simulink model "sampleModel7293_pp_1_1"  (R2018a)
settings: Solver=VariableStepAuto  StartTime=0.0  StopTime=10.0  RelTol=1e-3
undefined symbols (not defined in the file): DiscIntNeverNeededParam
libraries: simulink x367
(part 4 of 9)

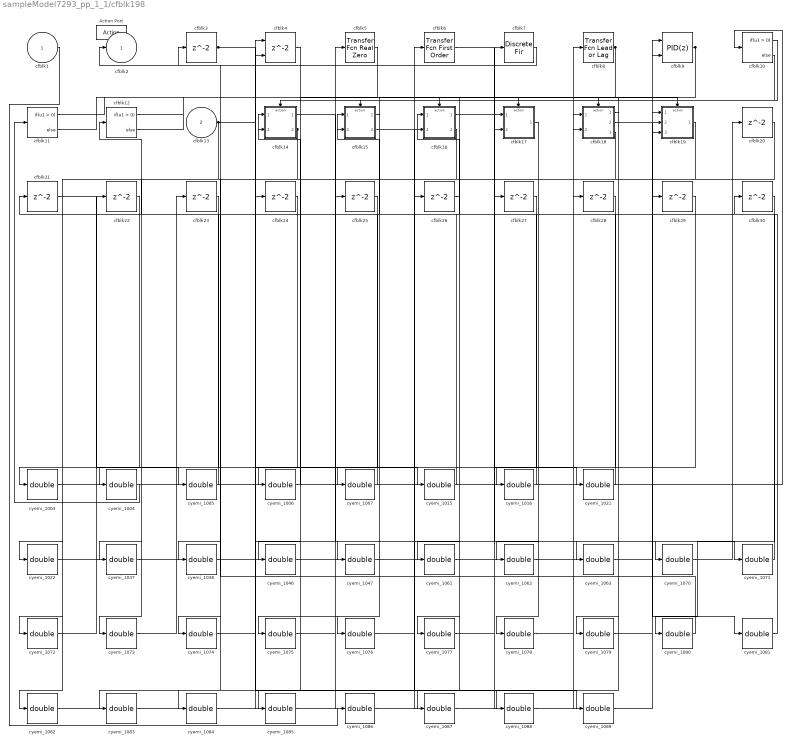
== system sampleModel7293_pp_1_1/cfblk198 ==
  cfblk1 : Inport
  cfblk13 : Inport  Port=2
  Action Port : ActionPort  ActionType=then
  cfblk10 : If  SampleTime=1
  cfblk11 : If  SampleTime=1
  cfblk12 : If  SampleTime=1
  cfblk14 : Subsystem  TreatAsAtomicUnit=on
  cfblk15 : Subsystem  TreatAsAtomicUnit=on
  cfblk16 : Subsystem  TreatAsAtomicUnit=on
  cfblk17 : Subsystem  TreatAsAtomicUnit=on
  cfblk18 : Subsystem  TreatAsAtomicUnit=on
  cfblk19 : Subsystem  TreatAsAtomicUnit=on
  cfblk{3,20..30} (12 alike) : Delay
  cfblk4 : Delay  ShowEnablePort=on
      settings: InputPortMap=u0,e6
  cfblk5 : simulink/Discrete/Transfer Fcn Real Zero  ZeroZ=0.75  ICPrevInput=0.0  DoSatur=off
      settings: SourceProductName=Simulink  SourceProductBaseCode=SL
  cfblk6 : simulink/Discrete/Transfer Fcn First Order  PoleZ=0.95  ICPrevOutput=0.0  DoSatur=off
      settings: SourceProductName=Simulink
  cfblk7 : DiscreteFir
  cfblk8 : simulink/Discrete/Transfer Fcn Lead or Lag  PoleZ=0.95  ZeroZ=0.75  ICPrevOutput=0.0  ICPrevInput=0.0  DoSatur=off
      settings: SourceProductName=Simulink  SourceProductBaseCode=SL
  cfblk9 : simulink/Continuous/PID Controller (2DOF)  Controller=PID  TimeDomain=Discrete-time  SampleTime=-1  IntegratorMethod=Forward Euler  FilterMethod=Forward Euler  Form=Parallel  UseFilter=on  ControllerParametersSource=internal  P=1  I=1  D=0  N=100  b=1  c=1  InitialConditionSource=internal  InitialConditionForIntegrator=0  InitialConditionForFilter=0  ExternalReset=none  LimitOutput=off  UpperSaturationLimit=inf  LowerSaturationLimit=-inf  LinearizeAsGain=off  AntiWindupMode=none  Kb=1  TrackingMode=off  Kt=1  PParamMin=[]  PParamMax=[]  IParamMin=[]  IParamMax=[]  DParamMin=[]  DParamMax=[]  NParamMin=[]  NParamMax=[]  bParamMin=[]  bParamMax=[]  cParamMin=[]  cParamMax=[]  KbParamMin=[]  KbParamMax=[]  KtParamMin=[]  KtParamMax=[]  POutMin=[]  POutMax=[]  IOutMin=[]  IOutMax=[]  DOutMin=[]  DOutMax=[]  NOutMin=[]  NOutMax=[]  bOutMin=[]  bOutMax=[]  cOutMin=[]  cOutMax=[]  KbOutMin=[]  KbOutMax=[]  KtOutMin=[]  KtOutMax=[]  IntegratorOutMin=[]  IntegratorOutMax=[]  FilterOutMin=[]  FilterOutMax=[]  SumOutMin=[]  SumOutMax=[]  Sum1OutMin=[]  Sum1OutMax=[]  Sum2OutMin=[]  Sum2OutMax=[]  Sum3OutMin=[]  Sum3OutMax=[]  SumI1OutMin=[]  SumI1OutMax=[]  SumI2OutMin=[]  SumI2OutMax=[]  SumI3OutMin=[]  SumI3OutMax=[]  SumDOutMin=[]  SumDOutMax=[]  SaturationOutMin=[]  SaturationOutMax=[]  IntegratorContinuousStateAttributes=''  IntegratorStateMustResolveToSignalObject=off  IntegratorRTWStateStorageClass=Auto  FilterContinuousStateAttributes=''  FilterStateMustResolveToSignalObject=off  FilterRTWStateStorageClass=Auto  DifferentiatorICPrevScaledInput=0  DifferentiatorOutMin=[]  DifferentiatorOutMax=[]  FilterDiffOutCoefMin=[]  FilterDiffOutCoefMax=[]  SumDenOutMin=[]  SumDenOutMax=[]  SumNumOutMin=[]  SumNumOutMax=[]  ReciprocalOutMin=[]  ReciprocalOutMax=[]  DivideOutMin=[]  DivideOutMax=[]  TunerSelectOption=Transfer Function Based (PID Tuner App)
  cyemi_{1003..1007,1015..1016,1021..1022,1037..1038,1046..1047,1061..1063,1070..1089} (36 alike) : DataTypeConversion  OutDataTypeStr=double
  cfblk2 : Outport
  wires:
  cfblk7/1 -> cfblk2/1
  cfblk3/1 -> cyemi_1047/1, cyemi_1063/1
  cfblk9/1 -> cyemi_1079/1, cyemi_1087/1
  cfblk13/1 -> cyemi_1004/1, cyemi_1015/1, cyemi_1089/1
  cfblk8/1 -> cyemi_1076/1, cyemi_1077/1
  cfblk14/2(cfblk11) -> cyemi_1073/1, cyemi_1074/1
  cfblk10/1 -> cfblk14/Action
  cfblk10/2 -> cfblk15/Action
  cfblk11/1 -> cfblk16/Action
  cfblk11/2 -> cfblk17/Action
  cfblk12/1 -> cfblk18/Action
  cfblk12/2 -> cfblk19/Action
  cyemi_1003/1 -> cfblk10/1
  cfblk24/1 -> cyemi_1003/1
  cyemi_1004/1 -> cfblk11/1
  cyemi_1005/1 -> cfblk12/1
  cfblk21/1 -> cyemi_1005/1
  cyemi_1006/1 -> cfblk14/1(cfblk1)
  cfblk5/1 -> cyemi_1006/1
  cyemi_1007/1 -> cfblk14/2(cfblk10)
  cfblk25/1 -> cyemi_1007/1
  cyemi_1015/1 -> cfblk15/1(cfblk1)
  cyemi_1016/1 -> cfblk15/2(cfblk6)
  cfblk29/1 -> cyemi_1016/1
  cyemi_1021/1 -> cfblk16/1(cfblk1)
  cfblk6/1 -> cyemi_1021/1
  cyemi_1022/1 -> cfblk16/2(cfblk14)
  cfblk23/1 -> cyemi_1022/1
  cyemi_1037/1 -> cfblk17/1(cfblk1)
  cfblk18/3(cfblk16) -> cyemi_1037/1
  cyemi_1038/1 -> cfblk17/2(cfblk10)
  cfblk27/1 -> cyemi_1038/1
  cyemi_1046/1 -> cfblk18/1(cfblk1)
  cfblk20/1 -> cyemi_1046/1
  cyemi_1047/1 -> cfblk18/2(cfblk14)
  cyemi_1061/1 -> cfblk19/1(cfblk1)
  cfblk26/1 -> cyemi_1061/1
  cyemi_1062/1 -> cfblk19/2(cfblk9)
  cfblk28/1 -> cyemi_1062/1
  cyemi_1063/1 -> cfblk19/3(cfblk10)
  cyemi_1070/1 -> cfblk20/1
  cfblk16/1(cfblk2) -> cyemi_1070/1
  cyemi_1071/1 -> cfblk21/1
  cfblk14/1(cfblk2) -> cyemi_1071/1
  cyemi_1072/1 -> cfblk22/1
  cfblk19/1(cfblk2) -> cyemi_1072/1
  cyemi_1073/1 -> cfblk23/1
  cyemi_1074/1 -> cfblk24/1
  cyemi_1075/1 -> cfblk25/1
  cfblk15/1(cfblk2) -> cyemi_1075/1
  cyemi_1076/1 -> cfblk26/1
  cyemi_1077/1 -> cfblk27/1
  cyemi_1078/1 -> cfblk28/1
  cfblk17/1(cfblk2) -> cyemi_1078/1
  cyemi_1079/1 -> cfblk29/1
  cyemi_1080/1 -> cfblk3/1
  cfblk30/1 -> cyemi_1080/1
  cyemi_1081/1 -> cfblk30/1
  cfblk18/2(cfblk15) -> cyemi_1081/1
  cyemi_1082/1 -> cfblk4/1
  cfblk22/1 -> cyemi_1082/1
  cyemi_1083/1 -> cfblk4/2
  cfblk18/1(cfblk2) -> cyemi_1083/1
  cyemi_1084/1 -> cfblk5/1
  cfblk16/2(cfblk15) -> cyemi_1084/1
  cyemi_1085/1 -> cfblk6/1
  cfblk4/1 -> cyemi_1085/1
  cyemi_1086/1 -> cfblk7/1
  cfblk1/1 -> cyemi_1086/1
  cyemi_1087/1 -> cfblk8/1
  cyemi_1088/1 -> cfblk9/1
  cfblk15/2(cfblk7) -> cyemi_1088/1
  cyemi_1089/1 -> cfblk9/2

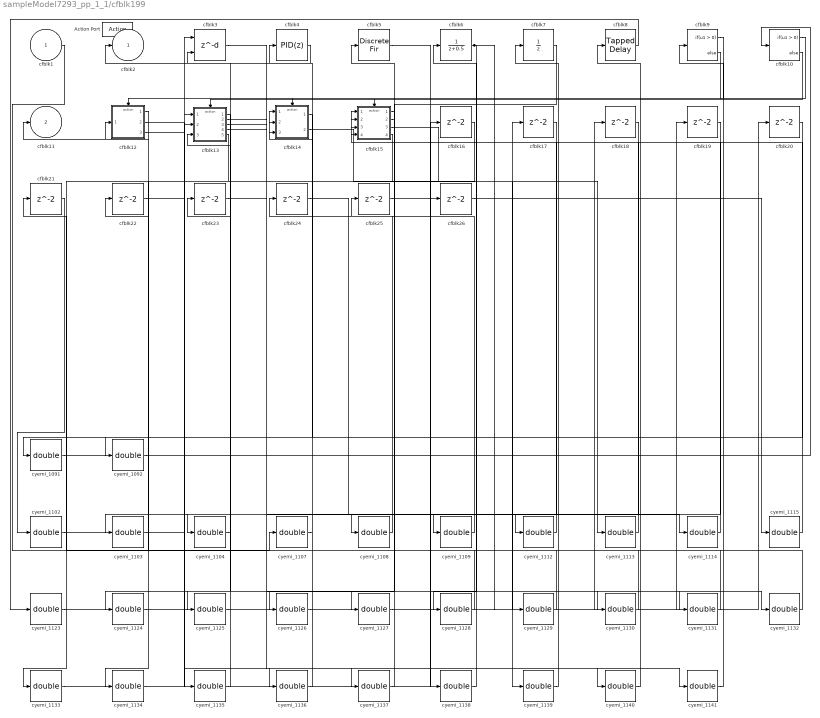
== system sampleModel7293_pp_1_1/cfblk199 ==
  cfblk1 : Inport
  Action Port : ActionPort  ActionType=else
  cfblk10 : If  SampleTime=1
  cfblk12 : Subsystem  TreatAsAtomicUnit=on
  cfblk13 : Subsystem  TreatAsAtomicUnit=on
  cfblk14 : Subsystem  TreatAsAtomicUnit=on
  cfblk15 : Subsystem  TreatAsAtomicUnit=on
  cfblk{16..26} (11 alike) : Delay
  cfblk3 : Delay  DelayLengthSource=Input port
      settings: InputPortMap=u0,p1
  cfblk4 : simulink/Continuous/PID Controller  Controller=PID  TimeDomain=Discrete-time  SampleTime=-1  IntegratorMethod=Forward Euler  FilterMethod=Forward Euler  Form=Parallel  UseFilter=on  ControllerParametersSource=internal  P=1  I=1  D=0  N=100  InitialConditionSource=internal  InitialConditionForIntegrator=0  InitialConditionForFilter=0  ExternalReset=none  LimitOutput=off  UpperSaturationLimit=inf  LowerSaturationLimit=-inf  LinearizeAsGain=off  AntiWindupMode=none  Kb=1  TrackingMode=off  Kt=1  PParamMin=[]  PParamMax=[]  IParamMin=[]  IParamMax=[]  DParamMin=[]  DParamMax=[]  NParamMin=[]  NParamMax=[]  KbParamMin=[]  KbParamMax=[]  KtParamMin=[]  KtParamMax=[]  POutMin=[]  POutMax=[]  IOutMin=[]  IOutMax=[]  DOutMin=[]  DOutMax=[]  NOutMin=[]  NOutMax=[]  KbOutMin=[]  KbOutMax=[]  KtOutMin=[]  KtOutMax=[]  IntegratorOutMin=[]  IntegratorOutMax=[]  FilterOutMin=[]  FilterOutMax=[]  SumOutMin=[]  SumOutMax=[]  SumI1OutMin=[]  SumI1OutMax=[]  SumI2OutMin=[]  SumI2OutMax=[]  SumI3OutMin=[]  SumI3OutMax=[]  SumDOutMin=[]  SumDOutMax=[]  SaturationOutMin=[]  SaturationOutMax=[]  IntegratorContinuousStateAttributes=''  IntegratorStateMustResolveToSignalObject=off  IntegratorRTWStateStorageClass=Auto  FilterContinuousStateAttributes=''  FilterStateMustResolveToSignalObject=off  FilterRTWStateStorageClass=Auto  DifferentiatorICPrevScaledInput=0  DifferentiatorOutMin=[]  DifferentiatorOutMax=[]  FilterDiffOutCoefMin=[]  FilterDiffOutCoefMax=[]  SumDenOutMin=[]  SumDenOutMax=[]  SumNumOutMin=[]  SumNumOutMax=[]  ReciprocalOutMin=[]  ReciprocalOutMax=[]  DivideOutMin=[]  DivideOutMax=[]  TunerSelectOption=Transfer Function Based (PID Tuner App)
  cfblk5 : DiscreteFir
  cfblk6 : DiscreteTransferFcn
  cfblk7 : UnitDelay  SampleTime=-1
  cfblk8 : simulink/Discrete/Tapped Delay  vinit=0.0  samptime=-1  NumDelays=1  DelayOrder=Oldest  includeCurrent=off
  cfblk9 : If  SampleTime=1
  cyemi_{1091..1092,1102..1104,1107..1109,1112..1115,1123..1141} (31 alike) : DataTypeConversion  OutDataTypeStr=double
  cfblk2 : Outport
  cfblk11 : Outport  Port=2
  wires:
  cfblk12/1(cfblk2) -> cfblk11/1
  cfblk6/1 -> cyemi_1128/1, cyemi_1129/1
  cfblk4/1 -> cfblk2/1
  cfblk9/1 -> cfblk12/Action
  cfblk9/2 -> cfblk13/Action
  cfblk10/1 -> cfblk14/Action
  cfblk10/2 -> cfblk15/Action
  cyemi_1091/1 -> cfblk10/1
  cfblk20/1 -> cyemi_1091/1
  cyemi_1092/1 -> cfblk12/1(cfblk1)
  cfblk14/1(cfblk2) -> cyemi_1092/1
  cyemi_1102/1 -> cfblk13/1(cfblk1)
  cfblk21/1 -> cyemi_1102/1
  cyemi_1103/1 -> cfblk13/2(cfblk5)
  cfblk18/1 -> cyemi_1103/1
  cyemi_1104/1 -> cfblk13/3(cfblk6)
  cfblk16/1 -> cyemi_1104/1
  cyemi_1107/1 -> cfblk14/1(cfblk1)
  cfblk1/1 -> cyemi_1107/1
  cyemi_1108/1 -> cfblk14/2(cfblk5)
  cfblk23/1 -> cyemi_1108/1
  cyemi_1109/1 -> cfblk14/3(cfblk6)
  cfblk19/1 -> cyemi_1109/1
  cyemi_1112/1 -> cfblk15/1(cfblk1)
  cfblk17/1 -> cyemi_1112/1
  cyemi_1113/1 -> cfblk15/2(cfblk9)
  cfblk14/2(cfblk7) -> cyemi_1113/1
  cyemi_1114/1 -> cfblk15/3(cfblk10)
  cfblk24/1 -> cyemi_1114/1
  cyemi_1115/1 -> cfblk15/4(cfblk11)
  cfblk26/1 -> cyemi_1115/1
  cyemi_1123/1 -> cfblk16/1
  cfblk8/1 -> cyemi_1123/1
  cyemi_1124/1 -> cfblk17/1
  cfblk13/1(cfblk2) -> cyemi_1124/1
  cyemi_1125/1 -> cfblk18/1
  cfblk15/1(cfblk2) -> cyemi_1125/1
  cyemi_1126/1 -> cfblk19/1
  cfblk15/2(cfblk12) -> cyemi_1126/1
  cyemi_1127/1 -> cfblk20/1
  cfblk7/1 -> cyemi_1127/1
  cyemi_1128/1 -> cfblk21/1
  cyemi_1129/1 -> cfblk22/1
  cyemi_1130/1 -> cfblk23/1
  cfblk13/2(cfblk7) -> cyemi_1130/1
  cyemi_1131/1 -> cfblk24/1
  cfblk13/3(cfblk8) -> cyemi_1131/1
  cyemi_1132/1 -> cfblk25/1
  cfblk13/4(cfblk9) -> cyemi_1132/1
  cyemi_1133/1 -> cfblk26/1
  cfblk13/5(cfblk10) -> cyemi_1133/1
  cyemi_1134/1 -> cfblk3/1
  cfblk15/4(cfblk14) -> cyemi_1134/1
  cyemi_1135/1 -> cfblk3/2
  cfblk22/1 -> cyemi_1135/1
  cyemi_1136/1 -> cfblk4/1
  cfblk12/2(cfblk9) -> cyemi_1136/1
  cyemi_1137/1 -> cfblk5/1
  cfblk3/1 -> cyemi_1137/1
  cyemi_1138/1 -> cfblk6/1
  cfblk5/1 -> cyemi_1138/1
  cyemi_1139/1 -> cfblk7/1
  cfblk15/3(cfblk13) -> cyemi_1139/1
  cyemi_1140/1 -> cfblk8/1
  cfblk12/3(cfblk10) -> cyemi_1140/1
  cyemi_1141/1 -> cfblk9/1
  cfblk25/1 -> cyemi_1141/1

== system sampleModel7293_pp_1_1/cfblk200 ==
  cfblk1 : Inport
  Action Port : ActionPort  ActionType=then
  cfblk10 : If  SampleTime=1
  cfblk11 : Subsystem  TreatAsAtomicUnit=on
  cfblk12 : Subsystem  TreatAsAtomicUnit=on
  cfblk13 : Delay
  cfblk14 : Delay
  cfblk3 : simulink/Discrete/Tapped Delay  vinit=0.0  samptime=-1  NumDelays=1  DelayOrder=Oldest  includeCurrent=off
  cfblk4 : simulink/Discrete/Difference  ICPrevInput=0.0  OutMin=[]  OutMax=[]  OutDataTypeStr=double  OutputDataTypeScalingMode=double  OutDataType=fixdt(1, 16)  OutScaling=2^-10  DoSatur=off
  cfblk5 : Delay  DelayLengthSource=Input port
      settings: InputPortMap=u0,p1
  cfblk6 : Delay
  cfblk7 : UnitDelay  SampleTime=-1
  cfblk8 : simulink/Continuous/PID Controller (2DOF)  Controller=PID  TimeDomain=Discrete-time  SampleTime=-1  IntegratorMethod=Forward Euler  FilterMethod=Forward Euler  Form=Parallel  UseFilter=on  ControllerParametersSource=internal  P=1  I=1  D=0  N=100  b=1  c=1  InitialConditionSource=internal  InitialConditionForIntegrator=0  InitialConditionForFilter=0  ExternalReset=none  LimitOutput=off  UpperSaturationLimit=inf  LowerSaturationLimit=-inf  LinearizeAsGain=off  AntiWindupMode=none  Kb=1  TrackingMode=off  Kt=1  PParamMin=[]  PParamMax=[]  IParamMin=[]  IParamMax=[]  DParamMin=[]  DParamMax=[]  NParamMin=[]  NParamMax=[]  bParamMin=[]  bParamMax=[]  cParamMin=[]  cParamMax=[]  KbParamMin=[]  KbParamMax=[]  KtParamMin=[]  KtParamMax=[]  POutMin=[]  POutMax=[]  IOutMin=[]  IOutMax=[]  DOutMin=[]  DOutMax=[]  NOutMin=[]  NOutMax=[]  bOutMin=[]  bOutMax=[]  cOutMin=[]  cOutMax=[]  KbOutMin=[]  KbOutMax=[]  KtOutMin=[]  KtOutMax=[]  IntegratorOutMin=[]  IntegratorOutMax=[]  FilterOutMin=[]  FilterOutMax=[]  SumOutMin=[]  SumOutMax=[]  Sum1OutMin=[]  Sum1OutMax=[]  Sum2OutMin=[]  Sum2OutMax=[]  Sum3OutMin=[]  Sum3OutMax=[]  SumI1OutMin=[]  SumI1OutMax=[]  SumI2OutMin=[]  SumI2OutMax=[]  SumI3OutMin=[]  SumI3OutMax=[]  SumDOutMin=[]  SumDOutMax=[]  SaturationOutMin=[]  SaturationOutMax=[]  IntegratorContinuousStateAttributes=''  IntegratorStateMustResolveToSignalObject=off  IntegratorRTWStateStorageClass=Auto  FilterContinuousStateAttributes=''  FilterStateMustResolveToSignalObject=off  FilterRTWStateStorageClass=Auto  DifferentiatorICPrevScaledInput=0  DifferentiatorOutMin=[]  DifferentiatorOutMax=[]  FilterDiffOutCoefMin=[]  FilterDiffOutCoefMax=[]  SumDenOutMin=[]  SumDenOutMax=[]  SumNumOutMin=[]  SumNumOutMax=[]  ReciprocalOutMin=[]  ReciprocalOutMax=[]  DivideOutMin=[]  DivideOutMax=[]  TunerSelectOption=Transfer Function Based (PID Tuner App)
  cfblk9 : UnitDelay  SampleTime=-1
  cyemi_{1145..1146,1157..1158,1169..1179} (15 alike) : DataTypeConversion  OutDataTypeStr=double
  cfblk2 : Outport
  wires:
  cfblk3/1 -> cyemi_1145/1, cyemi_1157/1, cyemi_1178/1
  cfblk9/1 -> cfblk2/1
  cfblk5/1 -> cyemi_1158/1, cyemi_1176/1
  cfblk6/1 -> cyemi_1174/1, cyemi_1179/1
  cfblk10/1 -> cfblk11/Action
  cfblk10/2 -> cfblk12/Action
  cyemi_1145/1 -> cfblk10/1
  cyemi_1146/1 -> cfblk11/1(cfblk1)
  cfblk14/1 -> cyemi_1146/1
  cyemi_1157/1 -> cfblk12/1(cfblk1)
  cyemi_1158/1 -> cfblk12/2(cfblk9)
  cyemi_1169/1 -> cfblk13/1
  cfblk8/1 -> cyemi_1169/1
  cyemi_1170/1 -> cfblk14/1
  cfblk4/1 -> cyemi_1170/1
  cyemi_1171/1 -> cfblk3/1
  cfblk7/1 -> cyemi_1171/1
  cyemi_1172/1 -> cfblk4/1
  cfblk11/1(cfblk2) -> cyemi_1172/1
  cyemi_1173/1 -> cfblk5/1
  cfblk13/1 -> cyemi_1173/1
  cyemi_1174/1 -> cfblk5/2
  cyemi_1175/1 -> cfblk6/1
  cfblk1/1 -> cyemi_1175/1
  cyemi_1176/1 -> cfblk7/1
  cyemi_1177/1 -> cfblk8/1
  cfblk12/1(cfblk2) -> cyemi_1177/1
  cyemi_1178/1 -> cfblk8/2
  cyemi_1179/1 -> cfblk9/1

== system sampleModel7293_pp_1_1/cfblk201 ==
  cfblk1 : Inport
  Action Port : ActionPort  ActionType=else
  cfblk10 : simulink/Discrete/Transfer Fcn First Order  PoleZ=0.95  ICPrevOutput=0.0  DoSatur=off
      settings: SourceProductName=Simulink
  cfblk11 : DiscreteIntegrator  SampleTime=-1  OutDataTypeStr=double  ICPrevOutput=DiscIntNeverNeededParam  ICPrevScaledInput=DiscIntNeverNeededParam
  cfblk12 : DiscreteTransferFcn
  cfblk13 : simulink/Discrete/Transfer Fcn Real Zero  ZeroZ=0.75  ICPrevInput=0.0  DoSatur=off
      settings: SourceProductName=Simulink  SourceProductBaseCode=SL
  cfblk14 : DiscreteStateSpace  SampleTime=-1
  cfblk15 : Delay
  cfblk3 : UnitDelay  SampleTime=-1
  cfblk4 : Delay  DelayLengthSource=Input port
      settings: InputPortMap=u0,p1
  cfblk5 : DiscreteFir
  cfblk6 : DiscreteTransferFcn
  cfblk7 : DiscreteIntegrator  SampleTime=-1  OutDataTypeStr=double  ICPrevOutput=DiscIntNeverNeededParam  ICPrevScaledInput=DiscIntNeverNeededParam
  cfblk8 : DiscreteStateSpace  SampleTime=-1
  cfblk9 : Delay
  cyemi_{1181..1194} (14 alike) : DataTypeConversion  OutDataTypeStr=double
  cfblk2 : Outport
  wires:
  cfblk1/1 -> cyemi_1189/1, cyemi_1190/1
  cfblk13/1 -> cfblk2/1
  cyemi_1181/1 -> cfblk10/1
  cfblk14/1 -> cyemi_1181/1
  cyemi_1182/1 -> cfblk11/1
  cfblk12/1 -> cyemi_1182/1
  cyemi_1183/1 -> cfblk12/1
  cfblk6/1 -> cyemi_1183/1
  cyemi_1184/1 -> cfblk13/1
  cfblk4/1 -> cyemi_1184/1
  cyemi_1185/1 -> cfblk14/1
  cfblk8/1 -> cyemi_1185/1
  cyemi_1186/1 -> cfblk15/1
  cfblk9/1 -> cyemi_1186/1
  cyemi_1187/1 -> cfblk3/1
  cfblk11/1 -> cyemi_1187/1
  cyemi_1188/1 -> cfblk4/1
  cfblk3/1 -> cyemi_1188/1
  cyemi_1189/1 -> cfblk4/2
  cyemi_1190/1 -> cfblk5/1
  cyemi_1191/1 -> cfblk6/1
  cfblk7/1 -> cyemi_1191/1
  cyemi_1192/1 -> cfblk7/1
  cfblk5/1 -> cyemi_1192/1
  cyemi_1193/1 -> cfblk8/1
  cfblk15/1 -> cyemi_1193/1
  cyemi_1194/1 -> cfblk9/1
  cfblk10/1 -> cyemi_1194/1

== system sampleModel7293_pp_1_1/cfblk202 ==
  cfblk1 : Inport
  Action Port : ActionPort  ActionType=then
  cfblk10 : DiscreteStateSpace  SampleTime=-1
  cfblk11 : DiscreteTransferFcn
  cfblk12 : Delay
  cfblk13 : Delay
  cfblk3 : simulink/Discrete/Tapped Delay  vinit=0.0  samptime=-1  NumDelays=1  DelayOrder=Oldest  includeCurrent=off
  cfblk4 : simulink/Discrete/Transfer Fcn Lead or Lag  PoleZ=0.95  ZeroZ=0.75  ICPrevOutput=0.0  ICPrevInput=0.0  DoSatur=off
      settings: SourceProductName=Simulink  SourceProductBaseCode=SL
  cfblk5 : simulink/Continuous/PID Controller (2DOF)  Controller=PID  TimeDomain=Discrete-time  SampleTime=-1  IntegratorMethod=Forward Euler  FilterMethod=Forward Euler  Form=Parallel  UseFilter=on  ControllerParametersSource=internal  P=1  I=1  D=0  N=100  b=1  c=1  InitialConditionSource=internal  InitialConditionForIntegrator=0  InitialConditionForFilter=0  ExternalReset=none  LimitOutput=off  UpperSaturationLimit=inf  LowerSaturationLimit=-inf  LinearizeAsGain=off  AntiWindupMode=none  Kb=1  TrackingMode=off  Kt=1  PParamMin=[]  PParamMax=[]  IParamMin=[]  IParamMax=[]  DParamMin=[]  DParamMax=[]  NParamMin=[]  NParamMax=[]  bParamMin=[]  bParamMax=[]  cParamMin=[]  cParamMax=[]  KbParamMin=[]  KbParamMax=[]  KtParamMin=[]  KtParamMax=[]  POutMin=[]  POutMax=[]  IOutMin=[]  IOutMax=[]  DOutMin=[]  DOutMax=[]  NOutMin=[]  NOutMax=[]  bOutMin=[]  bOutMax=[]  cOutMin=[]  cOutMax=[]  KbOutMin=[]  KbOutMax=[]  KtOutMin=[]  KtOutMax=[]  IntegratorOutMin=[]  IntegratorOutMax=[]  FilterOutMin=[]  FilterOutMax=[]  SumOutMin=[]  SumOutMax=[]  Sum1OutMin=[]  Sum1OutMax=[]  Sum2OutMin=[]  Sum2OutMax=[]  Sum3OutMin=[]  Sum3OutMax=[]  SumI1OutMin=[]  SumI1OutMax=[]  SumI2OutMin=[]  SumI2OutMax=[]  SumI3OutMin=[]  SumI3OutMax=[]  SumDOutMin=[]  SumDOutMax=[]  SaturationOutMin=[]  SaturationOutMax=[]  IntegratorContinuousStateAttributes=''  IntegratorStateMustResolveToSignalObject=off  IntegratorRTWStateStorageClass=Auto  FilterContinuousStateAttributes=''  FilterStateMustResolveToSignalObject=off  FilterRTWStateStorageClass=Auto  DifferentiatorICPrevScaledInput=0  DifferentiatorOutMin=[]  DifferentiatorOutMax=[]  FilterDiffOutCoefMin=[]  FilterDiffOutCoefMax=[]  SumDenOutMin=[]  SumDenOutMax=[]  SumNumOutMin=[]  SumNumOutMax=[]  ReciprocalOutMin=[]  ReciprocalOutMax=[]  DivideOutMin=[]  DivideOutMax=[]  TunerSelectOption=Transfer Function Based (PID Tuner App)
  cfblk6 : UnitDelay  SampleTime=-1
  cfblk7 : DiscreteFir
  cfblk8 : Delay  DelayLengthSource=Input port
      settings: InputPortMap=u0,p1
  cfblk9 : simulink/Continuous/PID Controller (2DOF)  Controller=PID  TimeDomain=Discrete-time  SampleTime=-1  IntegratorMethod=Forward Euler  FilterMethod=Forward Euler  Form=Parallel  UseFilter=on  ControllerParametersSource=internal  P=1  I=1  D=0  N=100  b=1  c=1  InitialConditionSource=internal  InitialConditionForIntegrator=0  InitialConditionForFilter=0  ExternalReset=none  LimitOutput=off  UpperSaturationLimit=inf  LowerSaturationLimit=-inf  LinearizeAsGain=off  AntiWindupMode=none  Kb=1  TrackingMode=off  Kt=1  PParamMin=[]  PParamMax=[]  IParamMin=[]  IParamMax=[]  DParamMin=[]  DParamMax=[]  NParamMin=[]  NParamMax=[]  bParamMin=[]  bParamMax=[]  cParamMin=[]  cParamMax=[]  KbParamMin=[]  KbParamMax=[]  KtParamMin=[]  KtParamMax=[]  POutMin=[]  POutMax=[]  IOutMin=[]  IOutMax=[]  DOutMin=[]  DOutMax=[]  NOutMin=[]  NOutMax=[]  bOutMin=[]  bOutMax=[]  cOutMin=[]  cOutMax=[]  KbOutMin=[]  KbOutMax=[]  KtOutMin=[]  KtOutMax=[]  IntegratorOutMin=[]  IntegratorOutMax=[]  FilterOutMin=[]  FilterOutMax=[]  SumOutMin=[]  SumOutMax=[]  Sum1OutMin=[]  Sum1OutMax=[]  Sum2OutMin=[]  Sum2OutMax=[]  Sum3OutMin=[]  Sum3OutMax=[]  SumI1OutMin=[]  SumI1OutMax=[]  SumI2OutMin=[]  SumI2OutMax=[]  SumI3OutMin=[]  SumI3OutMax=[]  SumDOutMin=[]  SumDOutMax=[]  SaturationOutMin=[]  SaturationOutMax=[]  IntegratorContinuousStateAttributes=''  IntegratorStateMustResolveToSignalObject=off  IntegratorRTWStateStorageClass=Auto  FilterContinuousStateAttributes=''  FilterStateMustResolveToSignalObject=off  FilterRTWStateStorageClass=Auto  DifferentiatorICPrevScaledInput=0  DifferentiatorOutMin=[]  DifferentiatorOutMax=[]  FilterDiffOutCoefMin=[]  FilterDiffOutCoefMax=[]  SumDenOutMin=[]  SumDenOutMax=[]  SumNumOutMin=[]  SumNumOutMax=[]  ReciprocalOutMin=[]  ReciprocalOutMax=[]  DivideOutMin=[]  DivideOutMax=[]  TunerSelectOption=Transfer Function Based (PID Tuner App)
  cyemi_{1196..1209} (14 alike) : DataTypeConversion  OutDataTypeStr=double
  cfblk2 : Outport
  wires:
  cfblk3/1 -> cyemi_1201/1, cyemi_1203/1, cyemi_1209/1
  cfblk9/1 -> cfblk2/1
  cfblk11/1 -> cyemi_1199/1, cyemi_1202/1
  cyemi_1196/1 -> cfblk10/1
  cfblk1/1 -> cyemi_1196/1
  cyemi_1197/1 -> cfblk11/1
  cfblk6/1 -> cyemi_1197/1
  cyemi_1198/1 -> cfblk12/1
  cfblk4/1 -> cyemi_1198/1
  cyemi_1199/1 -> cfblk13/1
  cyemi_1200/1 -> cfblk3/1
  cfblk12/1 -> cyemi_1200/1
  cyemi_1201/1 -> cfblk4/1
  cyemi_1202/1 -> cfblk5/1
  cyemi_1203/1 -> cfblk5/2
  cyemi_1204/1 -> cfblk6/1
  cfblk13/1 -> cyemi_1204/1
  cyemi_1205/1 -> cfblk7/1
  cfblk10/1 -> cyemi_1205/1
  cyemi_1206/1 -> cfblk8/1
  cfblk5/1 -> cyemi_1206/1
  cyemi_1207/1 -> cfblk8/2
  cfblk7/1 -> cyemi_1207/1
  cyemi_1208/1 -> cfblk9/1
  cfblk8/1 -> cyemi_1208/1
  cyemi_1209/1 -> cfblk9/2

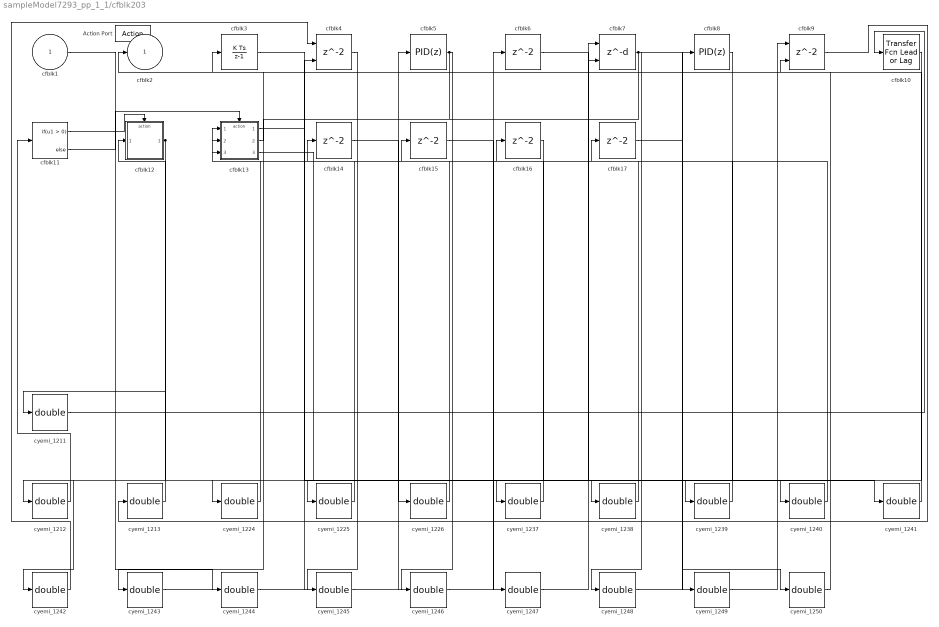
== system sampleModel7293_pp_1_1/cfblk203 ==
  cfblk1 : Inport
  Action Port : ActionPort  ActionType=else
  cfblk10 : simulink/Discrete/Transfer Fcn Lead or Lag  PoleZ=0.95  ZeroZ=0.75  ICPrevOutput=0.0  ICPrevInput=0.0  DoSatur=off
      settings: SourceProductName=Simulink  SourceProductBaseCode=SL
  cfblk11 : If  SampleTime=1
  cfblk12 : Subsystem  TreatAsAtomicUnit=on
  cfblk13 : Subsystem  TreatAsAtomicUnit=on
  cfblk{6,14..17} (5 alike) : Delay
  cfblk3 : DiscreteIntegrator  SampleTime=-1  OutDataTypeStr=double  ICPrevOutput=DiscIntNeverNeededParam  ICPrevScaledInput=DiscIntNeverNeededParam
  cfblk4 : Delay  ShowEnablePort=on
      settings: InputPortMap=u0,e6
  cfblk5 : simulink/Continuous/PID Controller  Controller=PID  TimeDomain=Discrete-time  SampleTime=-1  IntegratorMethod=Forward Euler  FilterMethod=Forward Euler  Form=Parallel  UseFilter=on  ControllerParametersSource=internal  P=1  I=1  D=0  N=100  InitialConditionSource=internal  InitialConditionForIntegrator=0  InitialConditionForFilter=0  ExternalReset=none  LimitOutput=off  UpperSaturationLimit=inf  LowerSaturationLimit=-inf  LinearizeAsGain=off  AntiWindupMode=none  Kb=1  TrackingMode=off  Kt=1  PParamMin=[]  PParamMax=[]  IParamMin=[]  IParamMax=[]  DParamMin=[]  DParamMax=[]  NParamMin=[]  NParamMax=[]  KbParamMin=[]  KbParamMax=[]  KtParamMin=[]  KtParamMax=[]  POutMin=[]  POutMax=[]  IOutMin=[]  IOutMax=[]  DOutMin=[]  DOutMax=[]  NOutMin=[]  NOutMax=[]  KbOutMin=[]  KbOutMax=[]  KtOutMin=[]  KtOutMax=[]  IntegratorOutMin=[]  IntegratorOutMax=[]  FilterOutMin=[]  FilterOutMax=[]  SumOutMin=[]  SumOutMax=[]  SumI1OutMin=[]  SumI1OutMax=[]  SumI2OutMin=[]  SumI2OutMax=[]  SumI3OutMin=[]  SumI3OutMax=[]  SumDOutMin=[]  SumDOutMax=[]  SaturationOutMin=[]  SaturationOutMax=[]  IntegratorContinuousStateAttributes=''  IntegratorStateMustResolveToSignalObject=off  IntegratorRTWStateStorageClass=Auto  FilterContinuousStateAttributes=''  FilterStateMustResolveToSignalObject=off  FilterRTWStateStorageClass=Auto  DifferentiatorICPrevScaledInput=0  DifferentiatorOutMin=[]  DifferentiatorOutMax=[]  FilterDiffOutCoefMin=[]  FilterDiffOutCoefMax=[]  SumDenOutMin=[]  SumDenOutMax=[]  SumNumOutMin=[]  SumNumOutMax=[]  ReciprocalOutMin=[]  ReciprocalOutMax=[]  DivideOutMin=[]  DivideOutMax=[]  TunerSelectOption=Transfer Function Based (PID Tuner App)
  cfblk7 : Delay  DelayLengthSource=Input port
      settings: InputPortMap=u0,p1
  cfblk8 : simulink/Continuous/PID Controller  Controller=PID  TimeDomain=Discrete-time  SampleTime=-1  IntegratorMethod=Forward Euler  FilterMethod=Forward Euler  Form=Parallel  UseFilter=on  ControllerParametersSource=internal  P=1  I=1  D=0  N=100  InitialConditionSource=internal  InitialConditionForIntegrator=0  InitialConditionForFilter=0  ExternalReset=none  LimitOutput=off  UpperSaturationLimit=inf  LowerSaturationLimit=-inf  LinearizeAsGain=off  AntiWindupMode=none  Kb=1  TrackingMode=off  Kt=1  PParamMin=[]  PParamMax=[]  IParamMin=[]  IParamMax=[]  DParamMin=[]  DParamMax=[]  NParamMin=[]  NParamMax=[]  KbParamMin=[]  KbParamMax=[]  KtParamMin=[]  KtParamMax=[]  POutMin=[]  POutMax=[]  IOutMin=[]  IOutMax=[]  DOutMin=[]  DOutMax=[]  NOutMin=[]  NOutMax=[]  KbOutMin=[]  KbOutMax=[]  KtOutMin=[]  KtOutMax=[]  IntegratorOutMin=[]  IntegratorOutMax=[]  FilterOutMin=[]  FilterOutMax=[]  SumOutMin=[]  SumOutMax=[]  SumI1OutMin=[]  SumI1OutMax=[]  SumI2OutMin=[]  SumI2OutMax=[]  SumI3OutMin=[]  SumI3OutMax=[]  SumDOutMin=[]  SumDOutMax=[]  SaturationOutMin=[]  SaturationOutMax=[]  IntegratorContinuousStateAttributes=''  IntegratorStateMustResolveToSignalObject=off  IntegratorRTWStateStorageClass=Auto  FilterContinuousStateAttributes=''  FilterStateMustResolveToSignalObject=off  FilterRTWStateStorageClass=Auto  DifferentiatorICPrevScaledInput=0  DifferentiatorOutMin=[]  DifferentiatorOutMax=[]  FilterDiffOutCoefMin=[]  FilterDiffOutCoefMax=[]  SumDenOutMin=[]  SumDenOutMax=[]  SumNumOutMin=[]  SumNumOutMax=[]  ReciprocalOutMin=[]  ReciprocalOutMax=[]  DivideOutMin=[]  DivideOutMax=[]  TunerSelectOption=Transfer Function Based (PID Tuner App)
  cfblk9 : Delay  ShowEnablePort=on
      settings: InputPortMap=u0,e6
  cyemi_{1211..1213,1224..1226,1237..1250} (20 alike) : DataTypeConversion  OutDataTypeStr=double
  cfblk2 : Outport
  wires:
  cfblk5/1 -> cyemi_1212/1, cyemi_1246/1
  cfblk12/1(cfblk2) -> cyemi_1211/1, cyemi_1242/1
  cfblk7/1 -> cyemi_1243/1, cyemi_1248/1, cyemi_1250/1
  cfblk13/2(cfblk14) -> cfblk2/1
  cfblk11/1 -> cfblk12/Action
  cfblk11/2 -> cfblk13/Action
  cyemi_1211/1 -> cfblk10/1
  cyemi_1212/1 -> cfblk11/1
  cyemi_1213/1 -> cfblk12/1(cfblk1)
  cfblk9/1 -> cyemi_1213/1
  cyemi_1224/1 -> cfblk13/1(cfblk1)
  cfblk16/1 -> cyemi_1224/1
  cyemi_1225/1 -> cfblk13/2(cfblk12)
  cfblk8/1 -> cyemi_1225/1
  cyemi_1226/1 -> cfblk13/3(cfblk13)
  cfblk14/1 -> cyemi_1226/1
  cyemi_1237/1 -> cfblk14/1
  cfblk3/1 -> cyemi_1237/1
  cyemi_1238/1 -> cfblk15/1
  cfblk13/3(cfblk15) -> cyemi_1238/1
  cyemi_1239/1 -> cfblk16/1
  cfblk10/1 -> cyemi_1239/1
  cyemi_1240/1 -> cfblk17/1
  cfblk6/1 -> cyemi_1240/1
  cyemi_1241/1 -> cfblk3/1
  cfblk13/1(cfblk2) -> cyemi_1241/1
  cyemi_1242/1 -> cfblk4/1
  cyemi_1243/1 -> cfblk4/2
  cyemi_1244/1 -> cfblk5/1
  cfblk1/1 -> cyemi_1244/1
  cyemi_1245/1 -> cfblk6/1
  cfblk4/1 -> cyemi_1245/1
  cyemi_1246/1 -> cfblk7/1
  cyemi_1247/1 -> cfblk7/2
  cfblk15/1 -> cyemi_1247/1
  cyemi_1248/1 -> cfblk8/1
  cyemi_1249/1 -> cfblk9/1
  cfblk17/1 -> cyemi_1249/1
  cyemi_1250/1 -> cfblk9/2

== system sampleModel7293_pp_1_1/cfblk204 ==
  cfblk1 : Inport
  cfblk11 : Inport  Port=2
  Action Port : ActionPort  ActionType=then
  cfblk10 : simulink/Discrete/Tapped Delay  vinit=0.0  samptime=-1  NumDelays=1  DelayOrder=Oldest  includeCurrent=off
  cfblk3 : simulink/Discrete/Transfer Fcn Real Zero  ZeroZ=0.75  ICPrevInput=0.0  DoSatur=off
      settings: SourceProductName=Simulink  SourceProductBaseCode=SL
  cfblk4 : simulink/Discrete/Transfer Fcn Lead or Lag  PoleZ=0.95  ZeroZ=0.75  ICPrevOutput=0.0  ICPrevInput=0.0  DoSatur=off
      settings: SourceProductName=Simulink  SourceProductBaseCode=SL
  cfblk5 : DiscreteZeroPole  Poles=[0 0.5]  Gain=1  SampleTime=-1
  cfblk6 : DiscreteZeroPole  Poles=[0 0.5]  Gain=1  SampleTime=-1
  cfblk7 : simulink/Discrete/Difference  ICPrevInput=0.0  OutMin=[]  OutMax=[]  OutDataTypeStr=double  OutputDataTypeScalingMode=double  OutDataType=fixdt(1, 16)  OutScaling=2^-10  DoSatur=off
  cfblk8 : simulink/Discrete/Transfer Fcn Real Zero  ZeroZ=0.75  ICPrevInput=0.0  DoSatur=off
      settings: SourceProductName=Simulink  SourceProductBaseCode=SL
  cfblk9 : DiscreteFilter
  cyemi_{1253..1260} (8 alike) : DataTypeConversion  OutDataTypeStr=double
  cfblk2 : Outport
  cfblk12 : Outport  Port=2
  cfblk13 : Outport  Port=3
  wires:
  cfblk8/1 -> cfblk2/1
  cfblk1/1 -> cfblk12/1
  cfblk6/1 -> cyemi_1254/1, cyemi_1258/1
  cfblk9/1 -> cfblk13/1
  cyemi_1253/1 -> cfblk10/1
  cfblk3/1 -> cyemi_1253/1
  cyemi_1254/1 -> cfblk3/1
  cyemi_1255/1 -> cfblk4/1
  cfblk10/1 -> cyemi_1255/1
  cyemi_1256/1 -> cfblk5/1
  cfblk7/1 -> cyemi_1256/1
  cyemi_1257/1 -> cfblk6/1
  cfblk11/1 -> cyemi_1257/1
  cyemi_1258/1 -> cfblk7/1
  cyemi_1259/1 -> cfblk8/1
  cfblk4/1 -> cyemi_1259/1
  cyemi_1260/1 -> cfblk9/1
  cfblk5/1 -> cyemi_1260/1

== system sampleModel7293_pp_1_1/cfblk205 ==
  cfblk1 : Inport
  cfblk9 : Inport  Port=2
  cfblk10 : Inport  Port=3
  Action Port : ActionPort  ActionType=else
  cfblk13 : Delay
  cfblk3 : DiscreteFir
  cfblk4 : simulink/Discrete/Transfer Fcn Lead or Lag  PoleZ=0.95  ZeroZ=0.75  ICPrevOutput=0.0  ICPrevInput=0.0  DoSatur=off
      settings: SourceProductName=Simulink  SourceProductBaseCode=SL
  cfblk5 : DiscreteZeroPole  Poles=[0 0.5]  Gain=1  SampleTime=-1
  cfblk6 : DiscreteFilter
  cfblk7 : simulink/Continuous/PID Controller (2DOF)  Controller=PID  TimeDomain=Discrete-time  SampleTime=-1  IntegratorMethod=Forward Euler  FilterMethod=Forward Euler  Form=Parallel  UseFilter=on  ControllerParametersSource=internal  P=1  I=1  D=0  N=100  b=1  c=1  InitialConditionSource=internal  InitialConditionForIntegrator=0  InitialConditionForFilter=0  ExternalReset=none  LimitOutput=off  UpperSaturationLimit=inf  LowerSaturationLimit=-inf  LinearizeAsGain=off  AntiWindupMode=none  Kb=1  TrackingMode=off  Kt=1  PParamMin=[]  PParamMax=[]  IParamMin=[]  IParamMax=[]  DParamMin=[]  DParamMax=[]  NParamMin=[]  NParamMax=[]  bParamMin=[]  bParamMax=[]  cParamMin=[]  cParamMax=[]  KbParamMin=[]  KbParamMax=[]  KtParamMin=[]  KtParamMax=[]  POutMin=[]  POutMax=[]  IOutMin=[]  IOutMax=[]  DOutMin=[]  DOutMax=[]  NOutMin=[]  NOutMax=[]  bOutMin=[]  bOutMax=[]  cOutMin=[]  cOutMax=[]  KbOutMin=[]  KbOutMax=[]  KtOutMin=[]  KtOutMax=[]  IntegratorOutMin=[]  IntegratorOutMax=[]  FilterOutMin=[]  FilterOutMax=[]  SumOutMin=[]  SumOutMax=[]  Sum1OutMin=[]  Sum1OutMax=[]  Sum2OutMin=[]  Sum2OutMax=[]  Sum3OutMin=[]  Sum3OutMax=[]  SumI1OutMin=[]  SumI1OutMax=[]  SumI2OutMin=[]  SumI2OutMax=[]  SumI3OutMin=[]  SumI3OutMax=[]  SumDOutMin=[]  SumDOutMax=[]  SaturationOutMin=[]  SaturationOutMax=[]  IntegratorContinuousStateAttributes=''  IntegratorStateMustResolveToSignalObject=off  IntegratorRTWStateStorageClass=Auto  FilterContinuousStateAttributes=''  FilterStateMustResolveToSignalObject=off  FilterRTWStateStorageClass=Auto  DifferentiatorICPrevScaledInput=0  DifferentiatorOutMin=[]  DifferentiatorOutMax=[]  FilterDiffOutCoefMin=[]  FilterDiffOutCoefMax=[]  SumDenOutMin=[]  SumDenOutMax=[]  SumNumOutMin=[]  SumNumOutMax=[]  ReciprocalOutMin=[]  ReciprocalOutMax=[]  DivideOutMin=[]  DivideOutMax=[]  TunerSelectOption=Transfer Function Based (PID Tuner App)
  cfblk8 : DiscreteFilter
  cyemi_{1264..1271} (8 alike) : DataTypeConversion  OutDataTypeStr=double
  cfblk2 : Outport
  cfblk11 : Outport  Port=2
  cfblk12 : Outport  Port=3
  wires:
  cfblk7/1 -> cyemi_1265/1, cyemi_1267/1
  cfblk9/1 -> cfblk12/1
  cfblk5/1 -> cfblk2/1
  cfblk8/1 -> cfblk11/1
  cyemi_1264/1 -> cfblk13/1
  cfblk3/1 -> cyemi_1264/1
  cyemi_1265/1 -> cfblk3/1
  cyemi_1266/1 -> cfblk4/1
  cfblk1/1 -> cyemi_1266/1
  cyemi_1267/1 -> cfblk5/1
  cyemi_1268/1 -> cfblk6/1
  cfblk10/1 -> cyemi_1268/1
  cyemi_1269/1 -> cfblk7/1
  cfblk4/1 -> cyemi_1269/1
  cyemi_1270/1 -> cfblk7/2
  cfblk13/1 -> cyemi_1270/1
  cyemi_1271/1 -> cfblk8/1
  cfblk6/1 -> cyemi_1271/1

== system sampleModel7293_pp_1_1/cfblk206 ==
  cfblk1 : Inport
  cfblk11 : Inport  Port=2
  cfblk12 : Inport  Port=3
  Action Port : ActionPort  ActionType=then
  cfblk10 : If  SampleTime=1
  cfblk16 : Subsystem  TreatAsAtomicUnit=on
  cfblk17 : Subsystem  TreatAsAtomicUnit=on
  cfblk{5,18..20} (4 alike) : Delay
  cfblk3 : simulink/Discrete/Difference  ICPrevInput=0.0  OutMin=[]  OutMax=[]  OutDataTypeStr=double  OutputDataTypeScalingMode=double  OutDataType=fixdt(1, 16)  OutScaling=2^-10  DoSatur=off
  cfblk4 : DiscreteIntegrator  SampleTime=-1  OutDataTypeStr=double  ICPrevOutput=DiscIntNeverNeededParam  ICPrevScaledInput=DiscIntNeverNeededParam
  cfblk6 : DiscreteStateSpace  SampleTime=-1
  cfblk7 : simulink/Discrete/Transfer Fcn First Order  PoleZ=0.95  ICPrevOutput=0.0  DoSatur=off
      settings: SourceProductName=Simulink
  cfblk8 : DiscreteTransferFcn
  cfblk9 : DiscreteTransferFcn
  cyemi_{1275..1277,1288..1289,1295..1304} (15 alike) : DataTypeConversion  OutDataTypeStr=double
  cfblk2 : Outport
  cfblk13 : Outport  Port=2
  cfblk14 : Outport  Port=3
  cfblk15 : Outport  Port=4
  wires:
  cfblk12/1 -> cfblk14/1
  cfblk6/1 -> cyemi_1303/1, cyemi_1304/1
  cfblk5/1 -> cfblk15/1
  cfblk16/2(cfblk13) -> cfblk13/1
  cfblk16/3(cfblk14) -> cfblk2/1
  cfblk17/1(cfblk2) -> cyemi_1295/1, cyemi_1301/1
  cfblk10/1 -> cfblk16/Action
  cfblk10/2 -> cfblk17/Action
  cyemi_1275/1 -> cfblk10/1
  cfblk18/1 -> cyemi_1275/1
  cyemi_1276/1 -> cfblk16/1(cfblk1)
  cfblk19/1 -> cyemi_1276/1
  cyemi_1277/1 -> cfblk16/2(cfblk12)
  cfblk11/1 -> cyemi_1277/1
  cyemi_1288/1 -> cfblk17/1(cfblk1)
  cfblk1/1 -> cyemi_1288/1
  cyemi_1289/1 -> cfblk17/2(cfblk7)
  cfblk20/1 -> cyemi_1289/1
  cyemi_1295/1 -> cfblk18/1
  cyemi_1296/1 -> cfblk19/1
  cfblk8/1 -> cyemi_1296/1
  cyemi_1297/1 -> cfblk20/1
  cfblk7/1 -> cyemi_1297/1
  cyemi_1298/1 -> cfblk3/1
  cfblk16/1(cfblk2) -> cyemi_1298/1
  cyemi_1299/1 -> cfblk4/1
  cfblk3/1 -> cyemi_1299/1
  cyemi_1300/1 -> cfblk5/1
  cfblk4/1 -> cyemi_1300/1
  cyemi_1301/1 -> cfblk6/1
  cyemi_1302/1 -> cfblk7/1
  cfblk9/1 -> cyemi_1302/1
  cyemi_1303/1 -> cfblk8/1
  cyemi_1304/1 -> cfblk9/1

== system sampleModel7293_pp_1_1/cfblk207 ==
  cfblk1 : Inport
  cfblk7 : Inport  Port=2
  Action Port : ActionPort  ActionType=else
  cfblk3 : simulink/Discrete/Transfer Fcn Real Zero  ZeroZ=0.75  ICPrevInput=0.0  DoSatur=off
      settings: SourceProductName=Simulink  SourceProductBaseCode=SL
  cfblk4 : simulink/Discrete/Transfer Fcn Lead or Lag  PoleZ=0.95  ZeroZ=0.75  ICPrevOutput=0.0  ICPrevInput=0.0  DoSatur=off
      settings: SourceProductName=Simulink  SourceProductBaseCode=SL
  cfblk5 : DiscreteFilter
  cfblk6 : UnitDelay  SampleTime=-1
  cyemi_{1307..1310} (4 alike) : DataTypeConversion  OutDataTypeStr=double
  cfblk2 : Outport
  wires:
  cfblk4/1 -> cfblk2/1
  cyemi_1307/1 -> cfblk3/1
  cfblk1/1 -> cyemi_1307/1
  cyemi_1308/1 -> cfblk4/1
  cfblk5/1 -> cyemi_1308/1
  cyemi_1309/1 -> cfblk5/1
  cfblk7/1 -> cyemi_1309/1
  cyemi_1310/1 -> cfblk6/1
  cfblk3/1 -> cyemi_1310/1

== system sampleModel7293_pp_1_1/cfblk208 ==
  cfblk1 : Inport
  cfblk12 : Inport  Port=2
  Action Port : ActionPort  ActionType=then
  cfblk10 : UnitDelay  SampleTime=-1
  cfblk11 : simulink/Discrete/Transfer Fcn Lead or Lag  PoleZ=0.95  ZeroZ=0.75  ICPrevOutput=0.0  ICPrevInput=0.0  DoSatur=off
      settings: SourceProductName=Simulink  SourceProductBaseCode=SL
  cfblk{8,14..16} (4 alike) : Delay
  cfblk3 : simulink/Continuous/PID Controller (2DOF)  Controller=PID  TimeDomain=Discrete-time  SampleTime=-1  IntegratorMethod=Forward Euler  FilterMethod=Forward Euler  Form=Parallel  UseFilter=on  ControllerParametersSource=internal  P=1  I=1  D=0  N=100  b=1  c=1  InitialConditionSource=internal  InitialConditionForIntegrator=0  InitialConditionForFilter=0  ExternalReset=none  LimitOutput=off  UpperSaturationLimit=inf  LowerSaturationLimit=-inf  LinearizeAsGain=off  AntiWindupMode=none  Kb=1  TrackingMode=off  Kt=1  PParamMin=[]  PParamMax=[]  IParamMin=[]  IParamMax=[]  DParamMin=[]  DParamMax=[]  NParamMin=[]  NParamMax=[]  bParamMin=[]  bParamMax=[]  cParamMin=[]  cParamMax=[]  KbParamMin=[]  KbParamMax=[]  KtParamMin=[]  KtParamMax=[]  POutMin=[]  POutMax=[]  IOutMin=[]  IOutMax=[]  DOutMin=[]  DOutMax=[]  NOutMin=[]  NOutMax=[]  bOutMin=[]  bOutMax=[]  cOutMin=[]  cOutMax=[]  KbOutMin=[]  KbOutMax=[]  KtOutMin=[]  KtOutMax=[]  IntegratorOutMin=[]  IntegratorOutMax=[]  FilterOutMin=[]  FilterOutMax=[]  SumOutMin=[]  SumOutMax=[]  Sum1OutMin=[]  Sum1OutMax=[]  Sum2OutMin=[]  Sum2OutMax=[]  Sum3OutMin=[]  Sum3OutMax=[]  SumI1OutMin=[]  SumI1OutMax=[]  SumI2OutMin=[]  SumI2OutMax=[]  SumI3OutMin=[]  SumI3OutMax=[]  SumDOutMin=[]  SumDOutMax=[]  SaturationOutMin=[]  SaturationOutMax=[]  IntegratorContinuousStateAttributes=''  IntegratorStateMustResolveToSignalObject=off  IntegratorRTWStateStorageClass=Auto  FilterContinuousStateAttributes=''  FilterStateMustResolveToSignalObject=off  FilterRTWStateStorageClass=Auto  DifferentiatorICPrevScaledInput=0  DifferentiatorOutMin=[]  DifferentiatorOutMax=[]  FilterDiffOutCoefMin=[]  FilterDiffOutCoefMax=[]  SumDenOutMin=[]  SumDenOutMax=[]  SumNumOutMin=[]  SumNumOutMax=[]  ReciprocalOutMin=[]  ReciprocalOutMax=[]  DivideOutMin=[]  DivideOutMax=[]  TunerSelectOption=Transfer Function Based (PID Tuner App)
  cfblk4 : UnitDelay  SampleTime=-1
  cfblk5 : DiscreteIntegrator  SampleTime=-1  OutDataTypeStr=double  ICPrevOutput=DiscIntNeverNeededParam  ICPrevScaledInput=DiscIntNeverNeededParam
  cfblk6 : DiscreteStateSpace  SampleTime=-1
  cfblk7 : simulink/Discrete/Transfer Fcn Lead or Lag  PoleZ=0.95  ZeroZ=0.75  ICPrevOutput=0.0  ICPrevInput=0.0  DoSatur=off
      settings: SourceProductName=Simulink  SourceProductBaseCode=SL
  cfblk9 : Delay  DelayLengthSource=Input port
      settings: InputPortMap=u0,p1
  cyemi_{1313..1326} (14 alike) : DataTypeConversion  OutDataTypeStr=double
  cfblk2 : Outport
  cfblk13 : Outport  Port=2
  wires:
  cfblk1/1 -> cfblk2/1
  cfblk9/1 -> cyemi_1316/1, cyemi_1321/1
  cfblk3/1 -> cfblk13/1, cyemi_1320/1
  cyemi_1313/1 -> cfblk10/1
  cfblk7/1 -> cyemi_1313/1
  cyemi_1314/1 -> cfblk11/1
  cfblk6/1 -> cyemi_1314/1
  cyemi_1315/1 -> cfblk14/1
  cfblk5/1 -> cyemi_1315/1
  cyemi_1316/1 -> cfblk15/1
  cyemi_1317/1 -> cfblk16/1
  cfblk11/1 -> cyemi_1317/1
  cyemi_1318/1 -> cfblk3/1
  cfblk14/1 -> cyemi_1318/1
  cyemi_1319/1 -> cfblk3/2
  cfblk15/1 -> cyemi_1319/1
  cyemi_1320/1 -> cfblk4/1
  cyemi_1321/1 -> cfblk5/1
  cyemi_1322/1 -> cfblk6/1
  cfblk16/1 -> cyemi_1322/1
  cyemi_1323/1 -> cfblk7/1
  cfblk4/1 -> cyemi_1323/1
  cyemi_1324/1 -> cfblk8/1
  cfblk12/1 -> cyemi_1324/1
  cyemi_1325/1 -> cfblk9/1
  cfblk8/1 -> cyemi_1325/1
  cyemi_1326/1 -> cfblk9/2
  cfblk10/1 -> cyemi_1326/1

== system sampleModel7293_pp_1_1/cfblk209 ==
  cfblk1 : Inport
  Action Port : ActionPort  ActionType=else
  cfblk10 : Subsystem  TreatAsAtomicUnit=on
  cfblk11 : Delay
  cfblk12 : Delay
  cfblk13 : Delay
  cfblk3 : DiscreteTransferFcn
  cfblk4 : DiscreteFir
  cfblk5 : simulink/Continuous/PID Controller (2DOF)  Controller=PID  TimeDomain=Discrete-time  SampleTime=-1  IntegratorMethod=Forward Euler  FilterMethod=Forward Euler  Form=Parallel  UseFilter=on  ControllerParametersSource=internal  P=1  I=1  D=0  N=100  b=1  c=1  InitialConditionSource=internal  InitialConditionForIntegrator=0  InitialConditionForFilter=0  ExternalReset=none  LimitOutput=off  UpperSaturationLimit=inf  LowerSaturationLimit=-inf  LinearizeAsGain=off  AntiWindupMode=none  Kb=1  TrackingMode=off  Kt=1  PParamMin=[]  PParamMax=[]  IParamMin=[]  IParamMax=[]  DParamMin=[]  DParamMax=[]  NParamMin=[]  NParamMax=[]  bParamMin=[]  bParamMax=[]  cParamMin=[]  cParamMax=[]  KbParamMin=[]  KbParamMax=[]  KtParamMin=[]  KtParamMax=[]  POutMin=[]  POutMax=[]  IOutMin=[]  IOutMax=[]  DOutMin=[]  DOutMax=[]  NOutMin=[]  NOutMax=[]  bOutMin=[]  bOutMax=[]  cOutMin=[]  cOutMax=[]  KbOutMin=[]  KbOutMax=[]  KtOutMin=[]  KtOutMax=[]  IntegratorOutMin=[]  IntegratorOutMax=[]  FilterOutMin=[]  FilterOutMax=[]  SumOutMin=[]  SumOutMax=[]  Sum1OutMin=[]  Sum1OutMax=[]  Sum2OutMin=[]  Sum2OutMax=[]  Sum3OutMin=[]  Sum3OutMax=[]  SumI1OutMin=[]  SumI1OutMax=[]  SumI2OutMin=[]  SumI2OutMax=[]  SumI3OutMin=[]  SumI3OutMax=[]  SumDOutMin=[]  SumDOutMax=[]  SaturationOutMin=[]  SaturationOutMax=[]  IntegratorContinuousStateAttributes=''  IntegratorStateMustResolveToSignalObject=off  IntegratorRTWStateStorageClass=Auto  FilterContinuousStateAttributes=''  FilterStateMustResolveToSignalObject=off  FilterRTWStateStorageClass=Auto  DifferentiatorICPrevScaledInput=0  DifferentiatorOutMin=[]  DifferentiatorOutMax=[]  FilterDiffOutCoefMin=[]  FilterDiffOutCoefMax=[]  SumDenOutMin=[]  SumDenOutMax=[]  SumNumOutMin=[]  SumNumOutMax=[]  ReciprocalOutMin=[]  ReciprocalOutMax=[]  DivideOutMin=[]  DivideOutMax=[]  TunerSelectOption=Transfer Function Based (PID Tuner App)
  cfblk6 : simulink/Discrete/Transfer Fcn Lead or Lag  PoleZ=0.95  ZeroZ=0.75  ICPrevOutput=0.0  ICPrevInput=0.0  DoSatur=off
      settings: SourceProductName=Simulink  SourceProductBaseCode=SL
  cfblk7 : simulink/Discrete/Difference  ICPrevInput=0.0  OutMin=[]  OutMax=[]  OutDataTypeStr=double  OutputDataTypeScalingMode=double  OutDataType=fixdt(1, 16)  OutScaling=2^-10  DoSatur=off
  cfblk8 : If  SampleTime=1
  cfblk9 : Subsystem  TreatAsAtomicUnit=on
  cyemi_{1328..1329,1341..1352} (14 alike) : DataTypeConversion  OutDataTypeStr=double
  cfblk2 : Outport
  wires:
  cfblk10/1(cfblk2) -> cfblk2/1
  cfblk7/1 -> cyemi_1342/1, cyemi_1343/1
  cfblk8/1 -> cfblk9/Action
  cfblk8/2 -> cfblk10/Action
  cyemi_1328/1 -> cfblk10/1(cfblk1)
  cfblk12/1 -> cyemi_1328/1
  cyemi_1329/1 -> cfblk10/2(cfblk12)
  cfblk13/1 -> cyemi_1329/1
  cyemi_1341/1 -> cfblk11/1
  cfblk5/1 -> cyemi_1341/1
  cyemi_1342/1 -> cfblk12/1
  cyemi_1343/1 -> cfblk13/1
  cyemi_1344/1 -> cfblk3/1
  cfblk9/1(cfblk2) -> cyemi_1344/1
  cyemi_1345/1 -> cfblk4/1
  cfblk6/1 -> cyemi_1345/1
  cyemi_1346/1 -> cfblk5/1
  cfblk3/1 -> cyemi_1346/1
  cyemi_1347/1 -> cfblk5/2
  cfblk9/2(cfblk16) -> cyemi_1347/1
  cyemi_1348/1 -> cfblk6/1
  cfblk1/1 -> cyemi_1348/1
  cyemi_1349/1 -> cfblk7/1
  cfblk10/3(cfblk14) -> cyemi_1349/1
  cyemi_1350/1 -> cfblk8/1
  cfblk4/1 -> cyemi_1350/1
  cyemi_1351/1 -> cfblk9/1(cfblk1)
  cfblk11/1 -> cyemi_1351/1
  cyemi_1352/1 -> cfblk9/2(cfblk15)
  cfblk10/2(cfblk13) -> cyemi_1352/1

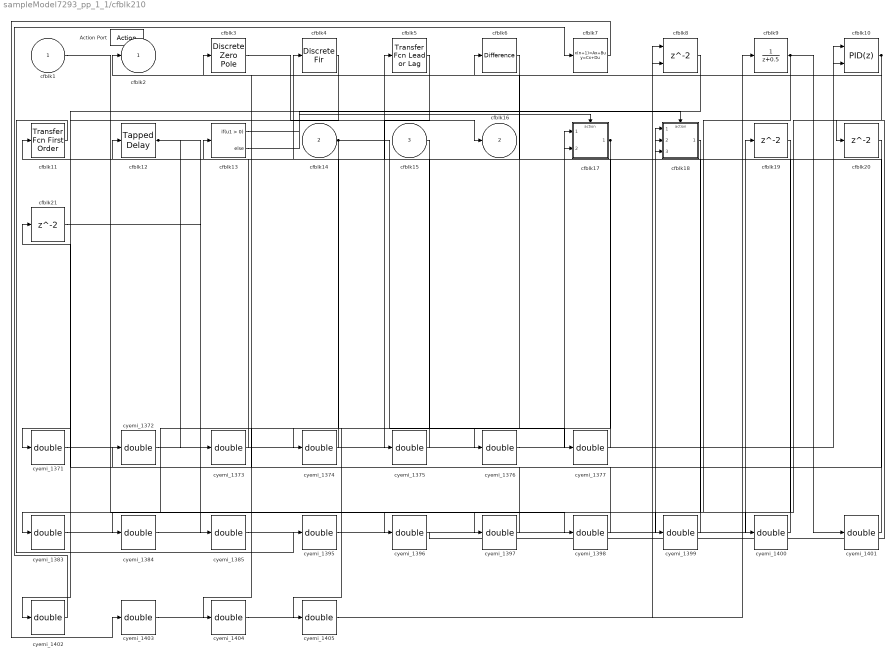
== system sampleModel7293_pp_1_1/cfblk210 ==
  cfblk1 : Inport
  cfblk14 : Inport  Port=2
  cfblk15 : Inport  Port=3
  Action Port : ActionPort  ActionType=then
  cfblk10 : simulink/Continuous/PID Controller (2DOF)  Controller=PID  TimeDomain=Discrete-time  SampleTime=-1  IntegratorMethod=Forward Euler  FilterMethod=Forward Euler  Form=Parallel  UseFilter=on  ControllerParametersSource=internal  P=1  I=1  D=0  N=100  b=1  c=1  InitialConditionSource=internal  InitialConditionForIntegrator=0  InitialConditionForFilter=0  ExternalReset=none  LimitOutput=off  UpperSaturationLimit=inf  LowerSaturationLimit=-inf  LinearizeAsGain=off  AntiWindupMode=none  Kb=1  TrackingMode=off  Kt=1  PParamMin=[]  PParamMax=[]  IParamMin=[]  IParamMax=[]  DParamMin=[]  DParamMax=[]  NParamMin=[]  NParamMax=[]  bParamMin=[]  bParamMax=[]  cParamMin=[]  cParamMax=[]  KbParamMin=[]  KbParamMax=[]  KtParamMin=[]  KtParamMax=[]  POutMin=[]  POutMax=[]  IOutMin=[]  IOutMax=[]  DOutMin=[]  DOutMax=[]  NOutMin=[]  NOutMax=[]  bOutMin=[]  bOutMax=[]  cOutMin=[]  cOutMax=[]  KbOutMin=[]  KbOutMax=[]  KtOutMin=[]  KtOutMax=[]  IntegratorOutMin=[]  IntegratorOutMax=[]  FilterOutMin=[]  FilterOutMax=[]  SumOutMin=[]  SumOutMax=[]  Sum1OutMin=[]  Sum1OutMax=[]  Sum2OutMin=[]  Sum2OutMax=[]  Sum3OutMin=[]  Sum3OutMax=[]  SumI1OutMin=[]  SumI1OutMax=[]  SumI2OutMin=[]  SumI2OutMax=[]  SumI3OutMin=[]  SumI3OutMax=[]  SumDOutMin=[]  SumDOutMax=[]  SaturationOutMin=[]  SaturationOutMax=[]  IntegratorContinuousStateAttributes=''  IntegratorStateMustResolveToSignalObject=off  IntegratorRTWStateStorageClass=Auto  FilterContinuousStateAttributes=''  FilterStateMustResolveToSignalObject=off  FilterRTWStateStorageClass=Auto  DifferentiatorICPrevScaledInput=0  DifferentiatorOutMin=[]  DifferentiatorOutMax=[]  FilterDiffOutCoefMin=[]  FilterDiffOutCoefMax=[]  SumDenOutMin=[]  SumDenOutMax=[]  SumNumOutMin=[]  SumNumOutMax=[]  ReciprocalOutMin=[]  ReciprocalOutMax=[]  DivideOutMin=[]  DivideOutMax=[]  TunerSelectOption=Transfer Function Based (PID Tuner App)
  cfblk11 : simulink/Discrete/Transfer Fcn First Order  PoleZ=0.95  ICPrevOutput=0.0  DoSatur=off
      settings: SourceProductName=Simulink
  cfblk12 : simulink/Discrete/Tapped Delay  vinit=0.0  samptime=-1  NumDelays=1  DelayOrder=Oldest  includeCurrent=off
  cfblk13 : If  SampleTime=1
  cfblk17 : Subsystem  TreatAsAtomicUnit=on
  cfblk18 : Subsystem  TreatAsAtomicUnit=on
  cfblk19 : Delay
  cfblk20 : Delay
  cfblk21 : Delay
  cfblk3 : DiscreteZeroPole  Poles=[0 0.5]  Gain=1  SampleTime=-1
  cfblk4 : DiscreteFir
  cfblk5 : simulink/Discrete/Transfer Fcn Lead or Lag  PoleZ=0.95  ZeroZ=0.75  ICPrevOutput=0.0  ICPrevInput=0.0  DoSatur=off
      settings: SourceProductName=Simulink  SourceProductBaseCode=SL
  cfblk6 : simulink/Discrete/Difference  ICPrevInput=0.0  OutMin=[]  OutMax=[]  OutDataTypeStr=double  OutputDataTypeScalingMode=double  OutDataType=fixdt(1, 16)  OutScaling=2^-10  DoSatur=off
  cfblk7 : DiscreteStateSpace  SampleTime=-1
  cfblk8 : Delay  ShowEnablePort=on
      settings: InputPortMap=u0,e6
  cfblk9 : DiscreteTransferFcn
  cyemi_{1371..1377,1383..1385,1395..1405} (21 alike) : DataTypeConversion  OutDataTypeStr=double
  cfblk2 : Outport
  cfblk16 : Outport  Port=2
  wires:
  cfblk14/1 -> cyemi_1377/1, cyemi_1404/1
  cfblk17/1(cfblk2) -> cyemi_1374/1, cyemi_1384/1
  cfblk10/1 -> cfblk2/1, cyemi_1400/1
  cfblk12/1 -> cyemi_1373/1, cyemi_1397/1
  cfblk9/1 -> cyemi_1399/1, cyemi_1401/1
  cfblk3/1 -> cfblk16/1
  cfblk13/1 -> cfblk17/Action
  cfblk13/2 -> cfblk18/Action
  cyemi_1371/1 -> cfblk10/1
  cfblk8/1 -> cyemi_1371/1
  cyemi_1372/1 -> cfblk10/2
  cfblk20/1 -> cyemi_1372/1
  cyemi_1373/1 -> cfblk11/1
  cyemi_1374/1 -> cfblk12/1
  cyemi_1375/1 -> cfblk13/1
  cfblk5/1 -> cyemi_1375/1
  cyemi_1376/1 -> cfblk17/1(cfblk1)
  cfblk6/1 -> cyemi_1376/1
  cyemi_1377/1 -> cfblk17/2(cfblk8)
  cyemi_1383/1 -> cfblk18/1(cfblk1)
  cfblk19/1 -> cyemi_1383/1
  cyemi_1384/1 -> cfblk18/2(cfblk12)
  cyemi_1385/1 -> cfblk18/3(cfblk13)
  cfblk21/1 -> cyemi_1385/1
  cyemi_1395/1 -> cfblk19/1
  cfblk11/1 -> cyemi_1395/1
  cyemi_1396/1 -> cfblk20/1
  cfblk18/1(cfblk2) -> cyemi_1396/1
  cyemi_1397/1 -> cfblk21/1
  cyemi_1398/1 -> cfblk3/1
  cfblk1/1 -> cyemi_1398/1
  cyemi_1399/1 -> cfblk4/1
  cyemi_1400/1 -> cfblk5/1
  cyemi_1401/1 -> cfblk6/1
  cyemi_1402/1 -> cfblk7/1
  cfblk4/1 -> cyemi_1402/1
  cyemi_1403/1 -> cfblk8/1
  cfblk7/1 -> cyemi_1403/1
  cyemi_1404/1 -> cfblk8/2
  cyemi_1405/1 -> cfblk9/1
  cfblk15/1 -> cyemi_1405/1

== system sampleModel7293_pp_1_1/cfblk211 ==
  cfblk1 : Inport
  Action Port : ActionPort  ActionType=else
  cfblk3 : DiscreteTransferFcn
  cfblk4 : Delay
  cfblk5 : simulink/Discrete/Transfer Fcn First Order  PoleZ=0.95  ICPrevOutput=0.0  DoSatur=off
      settings: SourceProductName=Simulink
  cfblk8 : Delay
  cyemi_{1407..1410} (4 alike) : DataTypeConversion  OutDataTypeStr=double
  cfblk2 : Outport
  cfblk6 : Outport  Port=2
  cfblk7 : Outport  Port=3
  wires:
  cfblk3/1 -> cfblk2/1
  cfblk1/1 -> cfblk6/1
  cfblk5/1 -> cfblk7/1, cyemi_1410/1
  cfblk4/1 -> cyemi_1407/1, cyemi_1409/1
  cyemi_1407/1 -> cfblk3/1
  cyemi_1408/1 -> cfblk4/1
  cfblk8/1 -> cyemi_1408/1
  cyemi_1409/1 -> cfblk5/1
  cyemi_1410/1 -> cfblk8/1

== system sampleModel7293_pp_1_1/cfblk212 ==
  cfblk1 : Inport
  cfblk8 : Inport  Port=2
  cfblk9 : Inport  Port=3
  Action Port : ActionPort  ActionType=then
  cfblk10 : Delay
  cfblk3 : Delay  ShowEnablePort=on
      settings: InputPortMap=u0,e6
  cfblk4 : simulink/Discrete/Transfer Fcn Lead or Lag  PoleZ=0.95  ZeroZ=0.75  ICPrevOutput=0.0  ICPrevInput=0.0  DoSatur=off
      settings: SourceProductName=Simulink  SourceProductBaseCode=SL
  cfblk5 : Delay
  cfblk6 : Delay  ShowEnablePort=on
      settings: InputPortMap=u0,e6
  cfblk7 : simulink/Continuous/PID Controller  Controller=PID  TimeDomain=Discrete-time  SampleTime=-1  IntegratorMethod=Forward Euler  FilterMethod=Forward Euler  Form=Parallel  UseFilter=on  ControllerParametersSource=internal  P=1  I=1  D=0  N=100  InitialConditionSource=internal  InitialConditionForIntegrator=0  InitialConditionForFilter=0  ExternalReset=none  LimitOutput=off  UpperSaturationLimit=inf  LowerSaturationLimit=-inf  LinearizeAsGain=off  AntiWindupMode=none  Kb=1  TrackingMode=off  Kt=1  PParamMin=[]  PParamMax=[]  IParamMin=[]  IParamMax=[]  DParamMin=[]  DParamMax=[]  NParamMin=[]  NParamMax=[]  KbParamMin=[]  KbParamMax=[]  KtParamMin=[]  KtParamMax=[]  POutMin=[]  POutMax=[]  IOutMin=[]  IOutMax=[]  DOutMin=[]  DOutMax=[]  NOutMin=[]  NOutMax=[]  KbOutMin=[]  KbOutMax=[]  KtOutMin=[]  KtOutMax=[]  IntegratorOutMin=[]  IntegratorOutMax=[]  FilterOutMin=[]  FilterOutMax=[]  SumOutMin=[]  SumOutMax=[]  SumI1OutMin=[]  SumI1OutMax=[]  SumI2OutMin=[]  SumI2OutMax=[]  SumI3OutMin=[]  SumI3OutMax=[]  SumDOutMin=[]  SumDOutMax=[]  SaturationOutMin=[]  SaturationOutMax=[]  IntegratorContinuousStateAttributes=''  IntegratorStateMustResolveToSignalObject=off  IntegratorRTWStateStorageClass=Auto  FilterContinuousStateAttributes=''  FilterStateMustResolveToSignalObject=off  FilterRTWStateStorageClass=Auto  DifferentiatorICPrevScaledInput=0  DifferentiatorOutMin=[]  DifferentiatorOutMax=[]  FilterDiffOutCoefMin=[]  FilterDiffOutCoefMax=[]  SumDenOutMin=[]  SumDenOutMax=[]  SumNumOutMin=[]  SumNumOutMax=[]  ReciprocalOutMin=[]  ReciprocalOutMax=[]  DivideOutMin=[]  DivideOutMax=[]  TunerSelectOption=Transfer Function Based (PID Tuner App)
  cyemi_{1414..1421} (8 alike) : DataTypeConversion  OutDataTypeStr=double
  cfblk2 : Outport
  wires:
  cfblk9/1 -> cfblk2/1
  cyemi_1414/1 -> cfblk10/1
  cfblk7/1 -> cyemi_1414/1
  cyemi_1415/1 -> cfblk3/1
  cfblk4/1 -> cyemi_1415/1
  cyemi_1416/1 -> cfblk3/2
  cfblk10/1 -> cyemi_1416/1
  cyemi_1417/1 -> cfblk4/1
  cfblk1/1 -> cyemi_1417/1
  cyemi_1418/1 -> cfblk5/1
  cfblk6/1 -> cyemi_1418/1
  cyemi_1419/1 -> cfblk6/1
  cfblk8/1 -> cyemi_1419/1
  cyemi_1420/1 -> cfblk6/2
  cfblk3/1 -> cyemi_1420/1
  cyemi_1421/1 -> cfblk7/1
  cfblk5/1 -> cyemi_1421/1
